simulink model "MIMO_FLOATING_POINT"  (R2023b)
settings: Solver=VariableStepAuto  StartTime=0.0  StopTime=1000  RelTol=1e-3
libraries: dspsigops x80, commchan3 x4, commdigbbndpm3 x2, commfilt2 x2, commsink2 x1, simulink x1, commrandsrc3 x1
(part 1 of 3)
settings Model: Creator=pc1  LastModifiedBy=yousi
settings SolverCC: AlgebraicLoopSolver=TrustRegion
settings DataIOCC: SaveOutput=off  SignalLogging=off  DSMLogging=off  SaveTime=off  ReturnWorkspaceOutputs=off
settings DebuggingCC: ArithmeticOperatorsInVariantConditions=warning
settings ModelReferenceCC: EnableRefExpFcnMdlSchedulingChecks=on
settings SFSimCC: CustomCodeUndefinedFunction=UseInterfaceOnly
settings CodeAppCC: StateflowObjectComments=on

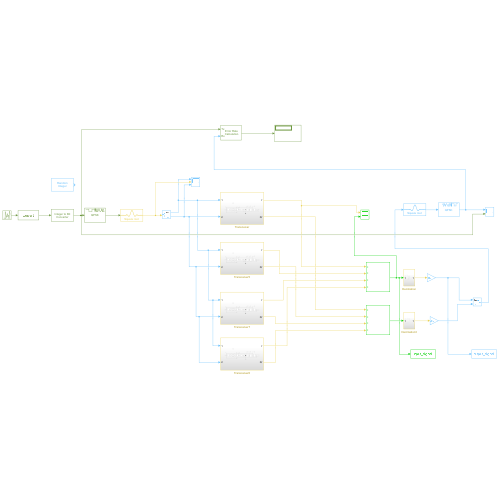
[thumbnail: Simulink's stored preview of the top-level diagram]
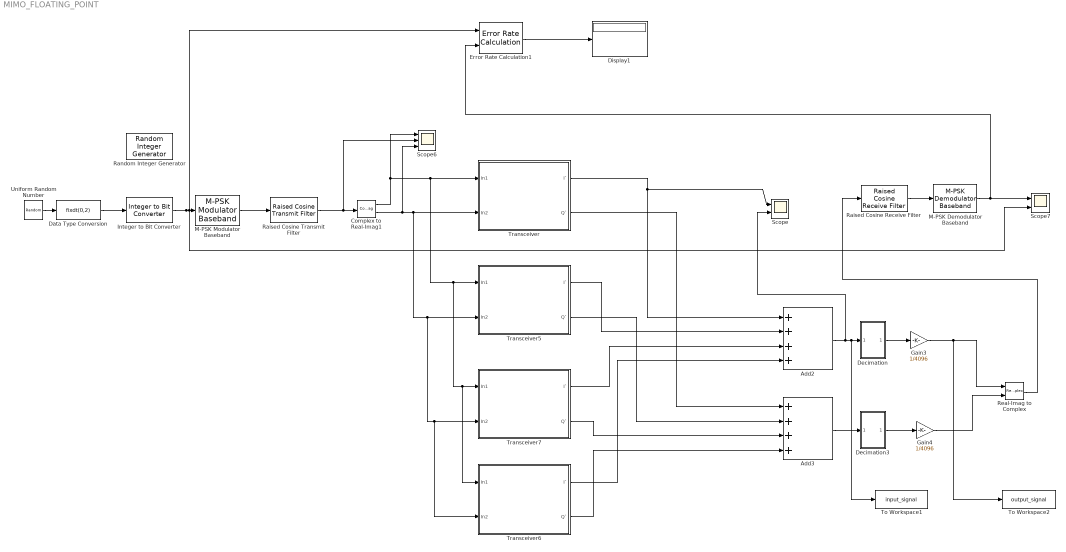
== system MIMO_FLOATING_POINT ==
  Add2 : Sum  Inputs=++++
  Add3 : Sum  Inputs=++++
  Complex to Real-Imag1 : ComplexToRealImag
  Data Type Conversion : DataTypeConversion  OutMin=0  OutMax=3  OutDataTypeStr=fixdt(0,2)  RndMeth=Round  SaturateOnIntegerOverflow=off
  Decimation : Subsystem
  Decimation3 : Subsystem
  Display1 : Display
  Error Rate Calculation1 : commsink2/Error Rate Calculation  N=28  st_delay=0  cp_mode=Entire frame  subframe=[]  PMode=Port  WsName=ErrorVec  RsMode2=off  stop=off  numErr=100  maxBits=1e6
  Gain3 : Gain  Gain=1/4096
  Gain4 : Gain  Gain=1/4096
  Integer to Bit Converter : simulink/Logic and Bit Operations/Integer to Bit Converter  nbits=2  signedInputValues=Unsigned  bitOrder=MSB first  outDtype=Inherit via internal rule
      settings: LibrarySourceBlock=|
      | commutil2/Integer to Bit
      | Converter
  M-PSK Demodulator Baseband : commdigbbndpm3/M-PSK Demodulator Baseband  M=4  OutType=Bit  DecType=Hard decision  VarSource=Dialog  Variance=1  Dec=Gray  Mapping=[0:7]  Ph=pi/4  outDtype1=Inherit via internal rule  outDtype2=Inherit via internal rule  derotateFactorWordLen=16  derotateFactorDataTypeStr=Inherit: Same word length as input  derotateFactorLastDataTypeStr=Inherit: Same word length as input
  M-PSK Modulator Baseband : commdigbbndpm3/M-PSK Modulator Baseband  M=4  InType=Bit  Enc=Gray  Mapping=[0:7]  Ph=pi/4  outDtype=double  outWordLen=16  outUDDataType=sfix(16)  outFracLenMode=Best precision  outFracLen=15  outDataTypeStr=double  outLastDataTypeStr=double
  Raised Cosine Receive Filter : commfilt2/Raised Cosine Receive Filter  filtType=Square root  R=0.35  filtSpan=8  N=2  downFactor=1  downOffset=0  filterGain=22  InputProcessing=Columns as channels (frame based)  RateOptions=Allow multirate processing  framing=Mute  checkCoeff=off  variableName=rcRxFilt  currentFiltSpan=10  D=5  inputOffset=0  sampMode=Mute  saveAsFlag=0  rateMode=Downsampling  checkGain=Normalized  launchFVT=on  roundingMode=Floor  overflowMode=off  coeffDataTypeStr=Inherit: Same word length as input  coeffMin=[]  coeffMax=[]  coeffLastDataTypeStr=Inherit: Same word length as input  accumDataTypeStr=Inherit: Same as product output  accumLastDataTypeStr=Inherit: Same as product output  outputDataTypeStr=Inherit: Same as accumulator  outputMin=[]  outputMax=[]  outputLastDataTypeStr=Inherit: Same as accumulator
  Raised Cosine Transmit Filter : commfilt2/Raised Cosine Transmit Filter  filtType=Square root  R=0.35  filtSpan=8  N=2  filterGain=22  InputProcessing=Columns as channels (frame based)  RateOptions=Allow multirate processing  framing=Mute  checkCoeff=off  variableName=rcTxFilt  checkGain=Normalized  sampMode=Mute  saveAsFlag=0  currentFiltSpan=10  D=5  launchFVT=on  roundingMode=Floor  overflowMode=off  coeffDataTypeStr=Inherit: Same word length as input  coeffMin=[]  coeffMax=[]  coeffLastDataTypeStr=Inherit: Same word length as input  outputDataTypeStr=Inherit: Same as accumulator  outputMin=[]  outputMax=[]  outputLastDataTypeStr=Inherit: Same as accumulator
  Random Integer Generator : commrandsrc3/Random Integer Generator  SetSize=2  SeedSource=Auto  Seed=0  SampleTime=0.64/4  SamplesPerFrame=2  OutputDataType=double  SimulateUsing=Interpreted execution
  Real-Imag to Complex : RealImagToComplex
  Scope : Scope  NumInputPorts=2
  Scope6 : Scope  NumInputPorts=3
  Scope7 : Scope  NumInputPorts=2
  To Workspace1 : ToWorkspace  VariableName=input_signal  SampleTime=-1
      settings: Save2DSignal=2-D array (concatenate along first dimension)
  To Workspace2 : ToWorkspace  VariableName=output_signal  SampleTime=-1
      settings: Save2DSignal=2-D array (concatenate along first dimension)
  Transceiver : Subsystem
  Transceiver5 : Subsystem
  Transceiver6 : Subsystem
  Transceiver7 : Subsystem
  Uniform Random Number : UniformRandomNumber  Minimum=0  Maximum=3  Seed=70  SampleTime=0.64
  wires:
  Integer to Bit Converter/1 -> Scope7/2, Error Rate Calculation1/1, M-PSK Modulator Baseband/1
  Gain3/1 -> To Workspace2/1, Real-Imag to Complex/1
  Transceiver/1(I`) -> Add2/1, Scope/1
  Raised Cosine Receive Filter/1 -> M-PSK Demodulator Baseband/1
  Add3/1 -> Decimation3/1(In1)
  Add2/1 -> Scope/2, To Workspace1/1, Decimation/1(In1)
  Transceiver6/2(Q`) -> Add3/4
  Transceiver6/1(I`) -> Add2/4
  Gain4/1 -> Real-Imag to Complex/2
  Transceiver7/1(I`) -> Add2/3
  Decimation3/1(Out1) -> Gain4/1
  Complex to Real-Imag1/1 -> Transceiver6/1(In1), Transceiver7/1(In1), Transceiver5/1(In1), Transceiver/1(In1), Scope6/1
  Uniform Random Number/1 -> Data Type Conversion/1
  Decimation/1(Out1) -> Gain3/1
  M-PSK Modulator Baseband/1 -> Raised Cosine Transmit Filter/1
  Transceiver5/2(Q`) -> Add3/2
  Transceiver/2(Q`) -> Add3/1
  Raised Cosine Transmit Filter/1 -> Complex to Real-Imag1/1, Scope6/2
  Transceiver5/1(I`) -> Add2/2
  Real-Imag to Complex/1 -> Raised Cosine Receive Filter/1
  M-PSK Demodulator Baseband/1 -> Scope7/1, Error Rate Calculation1/2
  Data Type Conversion/1 -> Integer to Bit Converter/1
  Complex to Real-Imag1/2 -> Transceiver6/2(In2), Transceiver7/2(In2), Transceiver5/2(In2), Transceiver/2(In2), Scope6/3
  Transceiver7/2(Q`) -> Add3/3
  Error Rate Calculation1/1 -> Display1/1

== system MIMO_FLOATING_POINT/Decimation ==
  In1 : Inport
  Add1 : Sum
  Delay{7..10,12..15} (8 alike) : Delay  DelayLength=1
  Downsample{,1..3,6..9} (8 alike) : DownSample  N=8  RateOptions=Allow multirate processing
  Downsample4 : DownSample  RateOptions=Allow multirate processing
  Downsample5 : DownSample  RateOptions=Allow multirate processing
  E0(Z)1 : Subsystem
  E1(Z)1 : Subsystem
  E10 : Subsystem
  E11 : Subsystem
  E12 : Subsystem
  E13 : Subsystem
  E14 : Subsystem
  E15 : Subsystem
  E8 : Subsystem
  E9 : Subsystem
  Gain1 : Gain  Gain=1/4096
  Sum3 : Sum  Inputs=|++++++++
  Out1 : Outport
  wires:
  Sum3/1 -> Gain1/1
  Downsample3/1 -> E11/1(In1)
  Delay7/1 -> Delay8/1, Downsample1/1
  Delay14/1 -> Delay15/1, Downsample8/1
  E13/1(Out1) -> Sum3/6
  E10/1(Out1) -> Sum3/3
  Downsample6/1 -> E12/1(In1)
  E14/1(Out1) -> Sum3/7
  E15/1(Out1) -> Sum3/8
  Delay9/1 -> Delay12/1, Downsample3/1
  E8/1(Out1) -> Sum3/1
  Delay10/1 -> Downsample5/1
  Downsample/1 -> E8/1(In1)
  Gain1/1 -> Downsample4/1, Delay10/1
  E11/1(Out1) -> Sum3/4
  Delay12/1 -> Delay13/1, Downsample6/1
  E9/1(Out1) -> Sum3/2
  In1/1 -> Delay7/1, Downsample/1
  Downsample8/1 -> E14/1(In1)
  E0(Z)1/1(Out1) -> Add1/1
  Delay13/1 -> Delay14/1, Downsample7/1
  Delay15/1 -> Downsample9/1
  Add1/1 -> Out1/1
  Downsample7/1 -> E13/1(In1)
  Delay8/1 -> Delay9/1, Downsample2/1
  Downsample2/1 -> E10/1(In1)
  Downsample4/1 -> E0(Z)1/1(Input)
  Downsample5/1 -> E1(Z)1/1(Input1)
  E12/1(Out1) -> Sum3/5
  E1(Z)1/1(Output) -> Add1/2
  Downsample1/1 -> E9/1(In1)
  Downsample9/1 -> E15/1(In1)

== system MIMO_FLOATING_POINT/Decimation3 ==
  In1 : Inport
  Add1 : Sum
  Delay{7..10,12..15} (8 alike) : Delay  DelayLength=1
  Downsample{,1..3,6..9} (8 alike) : DownSample  N=8  RateOptions=Allow multirate processing
  Downsample4 : DownSample  RateOptions=Allow multirate processing
  Downsample5 : DownSample  RateOptions=Allow multirate processing
  E0(Z)1 : Subsystem
  E1(Z)1 : Subsystem
  E10 : Subsystem
  E11 : Subsystem
  E12 : Subsystem
  E13 : Subsystem
  E14 : Subsystem
  E15 : Subsystem
  E8 : Subsystem
  E9 : Subsystem
  Gain1 : Gain  Gain=1/4096
  Sum3 : Sum  Inputs=|++++++++
  Out1 : Outport
  wires:
  Sum3/1 -> Gain1/1
  Downsample3/1 -> E11/1(In1)
  Delay7/1 -> Delay8/1, Downsample1/1
  Delay14/1 -> Delay15/1, Downsample8/1
  E13/1(Out1) -> Sum3/6
  E10/1(Out1) -> Sum3/3
  Downsample6/1 -> E12/1(In1)
  E14/1(Out1) -> Sum3/7
  E15/1(Out1) -> Sum3/8
  Delay9/1 -> Delay12/1, Downsample3/1
  E8/1(Out1) -> Sum3/1
  Delay10/1 -> Downsample5/1
  Downsample/1 -> E8/1(In1)
  Gain1/1 -> Downsample4/1, Delay10/1
  E11/1(Out1) -> Sum3/4
  Delay12/1 -> Delay13/1, Downsample6/1
  E9/1(Out1) -> Sum3/2
  In1/1 -> Delay7/1, Downsample/1
  Downsample8/1 -> E14/1(In1)
  E0(Z)1/1(Out1) -> Add1/1
  Delay13/1 -> Delay14/1, Downsample7/1
  Delay15/1 -> Downsample9/1
  Add1/1 -> Out1/1
  Downsample7/1 -> E13/1(In1)
  Delay8/1 -> Delay9/1, Downsample2/1
  Downsample2/1 -> E10/1(In1)
  Downsample4/1 -> E0(Z)1/1(Input)
  Downsample5/1 -> E1(Z)1/1(Input1)
  E12/1(Out1) -> Sum3/5
  E1(Z)1/1(Output) -> Add1/2
  Downsample1/1 -> E9/1(In1)
  Downsample9/1 -> E15/1(In1)

== system MIMO_FLOATING_POINT/Transceiver ==
  In1 : Inport
  In2 : Inport  Port=2
  ADC 1 : Subsystem
  AWGN Channel : commchan3/AWGN Channel  noiseMode="Signal to noise ratio  (SNR)"  EbNodB=10  EsNodB=10  SNRdB=22  bitsPerSym=1  Ps=1  Tsym=(1.000000e-02 * 1)  variance=0.0001  seed=67  InputProcessing=Columns as channels (frame based)
  CWM_RX2 : Subsystem
  CWM_TX_Chain_1 : Subsystem
  Constant2 : Constant  Value=0
  DDC2 : Subsystem
  DUC2 : Subsystem
  Gain : Gain  Gain=1/32
  Gain1 : Gain  Gain=1/256
  Gain2 : Gain  Gain=1/256
  Inter_Lever2 : Subsystem
  "Interpolation " : Subsystem
  Interpolation 1 : Subsystem
  Scope{,1..2,4,8} (5 alike) : Scope
  Scope3 : Scope  NumInputPorts=2
  Scope5 : Scope  NumInputPorts=2
  Sine Wave : Sin  Frequency=2*pi*25  Phase=pi/2  SampleTime=0.01*2
  Sine Wave1 : Sin  Frequency=2*pi*25  SampleTime=0.01*2
  Subsystem : Subsystem
  Subsystem1 : Subsystem
  I` : Outport
  Q` : Outport  Port=2
  wires:
  Inter_Lever2/2(EVEN_Q) -> DDC2/2(EVEN_Q)
  DUC2/1(Out2) -> Gain/1, Scope1/1
  CWM_TX_Chain_1/2(Q_1) -> Interpolation 1/1(Input)
  AWGN Channel/1 -> Scope3/1, ADC 1/1(In1)
  Constant2/1 -> CWM_TX_Chain_1/1(PHI), CWM_RX2/1(In1)
  Gain/1 -> AWGN Channel/1
  CWM_TX_Chain_1/1(I_1) -> "Interpolation "/1(Input)
  Inter_Lever2/1(ODD_I) -> DDC2/1(ODD_I), Scope4/1
  ADC 1/1(bits 1&0) -> Inter_Lever2/1(bits 1&0), Scope2/1, Scope3/2
  CWM_RX2/1(I`) -> Scope5/1, I`/1
  DDC2/1(I_DDC) -> CWM_RX2/2(I_DDC), Scope8/1
  DDC2/2(Q_DDC) -> CWM_RX2/3(Q_DDC)
  In1/1 -> CWM_TX_Chain_1/2(Processor_I), Scope5/2
  In2/1 -> CWM_TX_Chain_1/3(Processor_Q)
  Subsystem/1(Out1) -> DUC2/1(I_1), Scope/1
  Subsystem1/1(Out1) -> DUC2/2(Q_1)
  "Interpolation "/1(Out1) -> Gain1/1
  Interpolation 1/1(Out1) -> Gain2/1
  Gain1/1 -> Subsystem/1(In1)
  Gain2/1 -> Subsystem1/1(In1)
  CWM_RX2/2(Q`) -> Q`/1

== system MIMO_FLOATING_POINT/Transceiver5 ==
  In1 : Inport
  In2 : Inport  Port=2
  ADC 1 : Subsystem
  AWGN Channel : commchan3/AWGN Channel  noiseMode="Signal to noise ratio  (SNR)"  EbNodB=10  EsNodB=10  SNRdB=22  bitsPerSym=1  Ps=1  Tsym=(1.000000e-02 * 1)  variance=0.0001  seed=67  InputProcessing=Columns as channels (frame based)
  CWM_RX2 : Subsystem
  CWM_TX_Chain_1 : Subsystem
  Constant2 : Constant  Value=0.8131
  DDC2 : Subsystem
  DUC2 : Subsystem
  Gain : Gain  Gain=1/32
  Gain1 : Gain  Gain=1/256
  Gain2 : Gain  Gain=1/256
  Inter_Lever2 : Subsystem
  "Interpolation " : Subsystem
  Interpolation 1 : Subsystem
  Scope{,1..2,4,8} (5 alike) : Scope
  Scope3 : Scope  NumInputPorts=2
  Scope5 : Scope  NumInputPorts=2
  Sine Wave : Sin  Frequency=2*pi*25  Phase=pi/2  SampleTime=0.01*2
  Sine Wave1 : Sin  Frequency=2*pi*25  SampleTime=0.01*2
  Subsystem : Subsystem
  Subsystem1 : Subsystem
  I` : Outport
  Q` : Outport  Port=2
  wires:
  Inter_Lever2/2(EVEN_Q) -> DDC2/2(EVEN_Q)
  DUC2/1(Out2) -> Gain/1, Scope1/1
  CWM_TX_Chain_1/2(Q_1) -> Interpolation 1/1(Input)
  AWGN Channel/1 -> Scope3/1, ADC 1/1(In1)
  Constant2/1 -> CWM_TX_Chain_1/1(PHI), CWM_RX2/1(In1)
  Gain/1 -> AWGN Channel/1
  CWM_TX_Chain_1/1(I_1) -> "Interpolation "/1(Input)
  Inter_Lever2/1(ODD_I) -> DDC2/1(ODD_I), Scope4/1
  ADC 1/1(bits 1&0) -> Inter_Lever2/1(bits 1&0), Scope2/1, Scope3/2
  CWM_RX2/1(I`) -> Scope5/1, I`/1
  DDC2/1(I_DDC) -> CWM_RX2/2(I_DDC), Scope8/1
  DDC2/2(Q_DDC) -> CWM_RX2/3(Q_DDC)
  In1/1 -> CWM_TX_Chain_1/2(Processor_I), Scope5/2
  In2/1 -> CWM_TX_Chain_1/3(Processor_Q)
  Subsystem/1(Out1) -> DUC2/1(I_1), Scope/1
  Subsystem1/1(Out1) -> DUC2/2(Q_1)
  "Interpolation "/1(Out1) -> Gain1/1
  Interpolation 1/1(Out1) -> Gain2/1
  Gain1/1 -> Subsystem/1(In1)
  Gain2/1 -> Subsystem1/1(In1)
  CWM_RX2/2(Q`) -> Q`/1

== system MIMO_FLOATING_POINT/Transceiver6 ==
  In1 : Inport
  In2 : Inport  Port=2
  ADC 1 : Subsystem
  AWGN Channel : commchan3/AWGN Channel  noiseMode="Signal to noise ratio  (SNR)"  EbNodB=10  EsNodB=10  SNRdB=22  bitsPerSym=1  Ps=1  Tsym=(1.000000e-02 * 1)  variance=0.0001  seed=67  InputProcessing=Columns as channels (frame based)
  CWM_RX2 : Subsystem
  CWM_TX_Chain_1 : Subsystem
  Constant2 : Constant  Value=2.4393
  DDC2 : Subsystem
  DUC2 : Subsystem
  Gain : Gain  Gain=1/32
  Gain1 : Gain  Gain=1/256
  Gain2 : Gain  Gain=1/256
  Inter_Lever2 : Subsystem
  "Interpolation " : Subsystem
  Interpolation 1 : Subsystem
  Scope{,1..2,4,8} (5 alike) : Scope
  Scope3 : Scope  NumInputPorts=2
  Scope5 : Scope  NumInputPorts=2
  Sine Wave : Sin  Frequency=2*pi*25  Phase=pi/2  SampleTime=0.01*2
  Sine Wave1 : Sin  Frequency=2*pi*25  SampleTime=0.01*2
  Subsystem : Subsystem
  Subsystem1 : Subsystem
  I` : Outport
  Q` : Outport  Port=2
  wires:
  Inter_Lever2/2(EVEN_Q) -> DDC2/2(EVEN_Q)
  DUC2/1(Out2) -> Gain/1, Scope1/1
  CWM_TX_Chain_1/2(Q_1) -> Interpolation 1/1(Input)
  AWGN Channel/1 -> Scope3/1, ADC 1/1(In1)
  Constant2/1 -> CWM_TX_Chain_1/1(PHI), CWM_RX2/1(In1)
  Gain/1 -> AWGN Channel/1
  CWM_TX_Chain_1/1(I_1) -> "Interpolation "/1(Input)
  Inter_Lever2/1(ODD_I) -> DDC2/1(ODD_I), Scope4/1
  ADC 1/1(bits 1&0) -> Inter_Lever2/1(bits 1&0), Scope2/1, Scope3/2
  CWM_RX2/1(I`) -> Scope5/1, I`/1
  DDC2/1(I_DDC) -> CWM_RX2/2(I_DDC), Scope8/1
  DDC2/2(Q_DDC) -> CWM_RX2/3(Q_DDC)
  In1/1 -> CWM_TX_Chain_1/2(Processor_I), Scope5/2
  In2/1 -> CWM_TX_Chain_1/3(Processor_Q)
  Subsystem/1(Out1) -> DUC2/1(I_1), Scope/1
  Subsystem1/1(Out1) -> DUC2/2(Q_1)
  "Interpolation "/1(Out1) -> Gain1/1
  Interpolation 1/1(Out1) -> Gain2/1
  Gain1/1 -> Subsystem/1(In1)
  Gain2/1 -> Subsystem1/1(In1)
  CWM_RX2/2(Q`) -> Q`/1

== system MIMO_FLOATING_POINT/Transceiver7 ==
  In1 : Inport
  In2 : Inport  Port=2
  ADC 1 : Subsystem
  AWGN Channel : commchan3/AWGN Channel  noiseMode="Signal to noise ratio  (SNR)"  EbNodB=10  EsNodB=10  SNRdB=22  bitsPerSym=1  Ps=1  Tsym=(1.000000e-02 * 1)  variance=0.0001  seed=67  InputProcessing=Columns as channels (frame based)
  CWM_RX2 : Subsystem
  CWM_TX_Chain_1 : Subsystem
  Constant2 : Constant  Value=1.6262
  DDC2 : Subsystem
  DUC2 : Subsystem
  Gain : Gain  Gain=1/32
  Gain1 : Gain  Gain=1/256
  Gain2 : Gain  Gain=1/256
  Inter_Lever2 : Subsystem
  "Interpolation " : Subsystem
  Interpolation 1 : Subsystem
  Scope{,1..2,4,8} (5 alike) : Scope
  Scope3 : Scope  NumInputPorts=2
  Scope5 : Scope  NumInputPorts=2
  Sine Wave : Sin  Frequency=2*pi*25  Phase=pi/2  SampleTime=0.01*2
  Sine Wave1 : Sin  Frequency=2*pi*25  SampleTime=0.01*2
  Subsystem : Subsystem
  Subsystem1 : Subsystem
  I` : Outport
  Q` : Outport  Port=2
  wires:
  Inter_Lever2/2(EVEN_Q) -> DDC2/2(EVEN_Q)
  DUC2/1(Out2) -> Gain/1, Scope1/1
  CWM_TX_Chain_1/2(Q_1) -> Interpolation 1/1(Input)
  AWGN Channel/1 -> Scope3/1, ADC 1/1(In1)
  Constant2/1 -> CWM_TX_Chain_1/1(PHI), CWM_RX2/1(In1)
  Gain/1 -> AWGN Channel/1
  CWM_TX_Chain_1/1(I_1) -> "Interpolation "/1(Input)
  Inter_Lever2/1(ODD_I) -> DDC2/1(ODD_I), Scope4/1
  ADC 1/1(bits 1&0) -> Inter_Lever2/1(bits 1&0), Scope2/1, Scope3/2
  CWM_RX2/1(I`) -> Scope5/1, I`/1
  DDC2/1(I_DDC) -> CWM_RX2/2(I_DDC), Scope8/1
  DDC2/2(Q_DDC) -> CWM_RX2/3(Q_DDC)
  In1/1 -> CWM_TX_Chain_1/2(Processor_I), Scope5/2
  In2/1 -> CWM_TX_Chain_1/3(Processor_Q)
  Subsystem/1(Out1) -> DUC2/1(I_1), Scope/1
  Subsystem1/1(Out1) -> DUC2/2(Q_1)
  "Interpolation "/1(Out1) -> Gain1/1
  Interpolation 1/1(Out1) -> Gain2/1
  Gain1/1 -> Subsystem/1(In1)
  Gain2/1 -> Subsystem1/1(In1)
  CWM_RX2/2(Q`) -> Q`/1

== system MIMO_FLOATING_POINT/Decimation/E0(Z)1 ==
  Input : Inport
  Delay : Delay  DelayLength=5
  Gain : Gain  Gain=0.5
  Out1 : Outport
  wires:
  Input/1 -> Gain/1
  Delay/1 -> Out1/1
  Gain/1 -> Delay/1

== system MIMO_FLOATING_POINT/Decimation/E1(Z)1 ==
  Input1 : Inport
  10-12 : Gain  Gain=0.3078
  2-20 : Gain  Gain=0.0011
  4-18 : Gain  Gain=-0.0072
  6-16 : Gain  Gain=0.0263
  8-14 : Gain  Gain=-0.078
  Add{7..10,12..16} (9 alike) : Sum
  Delay{21,23,25,27,29,31,33,35,37} (9 alike) : Delay  DelayLength=1
  Output : Outport
  wires:
  8-14/1 -> Add13/1, Add9/1
  Delay29/1 -> Add12/2  "x[n-11]"
  Add14/1 -> Delay35/1
  Input1/1 -> 2-20/1, 4-18/1, 6-16/1, 8-14/1, 10-12/1
  Add8/1 -> Delay25/1
  4-18/1 -> Add15/1, Add7/1
  Delay33/1 -> Add14/2  "x[n-15]"
  Add12/1 -> Delay31/1
  10-12/1 -> Add10/1, Add12/1
  Add9/1 -> Delay27/1
  Add16/1 -> Output/1
  Delay37/1 -> Add16/2  "x[n-19]"
  6-16/1 -> Add14/1, Add8/1
  Delay25/1 -> Add9/2  "x[n-7]"
  Add7/1 -> Delay23/1
  Add15/1 -> Delay37/1
  Delay23/1 -> Add8/2  "x[n-5]"
  Delay27/1 -> Add10/2  "x[n-9]"
  Delay31/1 -> Add13/2  "x[n-13]"
  Delay35/1 -> Add15/2  "x[n-17]"
  Delay21/1 -> Add7/2  "x[n-3]"
  2-20/1 -> Delay21/1, Add16/1
  Add13/1 -> Delay33/1
  Add10/1 -> Delay29/1

== system MIMO_FLOATING_POINT/Decimation/E10 ==
  In1 : Inport
  Delay3 : Delay  DelayLength=1
  Delay4 : Delay  DelayLength=1
  Delay5 : Delay  DelayLength=1
  Gain : Gain  Gain=10
  Gain1 : Gain  Gain=246
  Sum : Sum
  Sum1 : Sum
  Sum2 : Sum
  Out1 : Outport
  wires:
  In1/1 -> Gain1/1, Gain/1
  Sum1/1 -> Delay5/1
  Sum/1 -> Delay4/1
  Gain1/1 -> Sum1/1, Sum/1
  Delay3/1 -> Sum/2
  Delay4/1 -> Sum1/2
  Gain/1 -> Sum2/1, Delay3/1
  Delay5/1 -> Sum2/2
  Sum2/1 -> Out1/1

== system MIMO_FLOATING_POINT/Decimation/E11 ==
  In1 : Inport
  Delay3 : Delay  DelayLength=1
  Delay4 : Delay  DelayLength=1
  Delay5 : Delay  DelayLength=1
  Gain : Gain  Gain=4
  Gain1 : Gain  Gain=204
  Gain2 : Gain  Gain=284
  Gain3 : Gain  Gain=20
  Sum : Sum
  Sum1 : Sum
  Sum2 : Sum
  Out1 : Outport
  wires:
  In1/1 -> Gain2/1, Gain3/1, Gain1/1, Gain/1
  Sum1/1 -> Delay5/1
  Sum/1 -> Delay4/1
  Gain1/1 -> Sum/1
  Delay3/1 -> Sum/2
  Delay4/1 -> Sum1/2
  Gain3/1 -> Sum2/1
  Delay5/1 -> Sum2/2
  Gain/1 -> Delay3/1
  Sum2/1 -> Out1/1
  Gain2/1 -> Sum1/1

== system MIMO_FLOATING_POINT/Decimation/E12 ==
  In1 : Inport
  Delay3 : Delay  DelayLength=1
  Delay4 : Delay  DelayLength=1
  Delay5 : Delay  DelayLength=1
  Gain : Gain
  Gain1 : Gain  Gain=161
  Gain2 : Gain  Gain=315
  Gain3 : Gain  Gain=35
  Sum : Sum
  Sum1 : Sum
  Sum2 : Sum
  Out1 : Outport
  wires:
  In1/1 -> Gain2/1, Gain3/1, Gain1/1, Gain/1
  Sum1/1 -> Delay5/1
  Sum/1 -> Delay4/1
  Gain1/1 -> Sum/1
  Delay3/1 -> Sum/2
  Delay4/1 -> Sum1/2
  Gain3/1 -> Sum2/1
  Delay5/1 -> Sum2/2
  Gain/1 -> Delay3/1
  Sum2/1 -> Out1/1
  Gain2/1 -> Sum1/1

== system MIMO_FLOATING_POINT/Decimation/E13 ==
  In1 : Inport
  Delay6 : Delay  DelayLength=1
  Delay7 : Delay  DelayLength=1
  Gain4 : Gain  Gain=120
  Gain5 : Gain  Gain=336
  Gain6 : Gain  Gain=56
  Sum4 : Sum
  Sum5 : Sum
  Out1 : Outport
  wires:
  Gain4/1 -> Delay6/1
  In1/1 -> Gain6/1, Gain5/1, Gain4/1
  Sum5/1 -> Out1/1
  Sum4/1 -> Delay7/1
  Delay7/1 -> Sum5/2
  Gain6/1 -> Sum5/1
  Gain5/1 -> Sum4/1
  Delay6/1 -> Sum4/2

== system MIMO_FLOATING_POINT/Decimation/E14 ==
  In1 : Inport
  Delay6 : Delay  DelayLength=1
  Delay7 : Delay  DelayLength=1
  Gain4 : Gain  Gain=84
  Gain5 : Gain  Gain=344
  Sum4 : Sum
  Sum5 : Sum
  Out1 : Outport
  wires:
  In1/1 -> Gain5/1, Gain4/1
  Sum5/1 -> Out1/1
  Sum4/1 -> Delay7/1
  Delay7/1 -> Sum5/2
  Gain4/1 -> Sum5/1, Delay6/1
  Gain5/1 -> Sum4/1
  Delay6/1 -> Sum4/2

== system MIMO_FLOATING_POINT/Decimation/E15 ==
  In1 : Inport
  Delay6 : Delay  DelayLength=1
  Delay7 : Delay  DelayLength=1
  Gain4 : Gain  Gain=56
  Gain5 : Gain  Gain=336
  Gain6 : Gain  Gain=120
  Sum4 : Sum
  Sum5 : Sum
  Out1 : Outport
  wires:
  Gain4/1 -> Delay6/1
  In1/1 -> Gain6/1, Gain5/1, Gain4/1
  Sum5/1 -> Out1/1
  Sum4/1 -> Delay7/1
  Delay7/1 -> Sum5/2
  Gain6/1 -> Sum5/1
  Gain5/1 -> Sum4/1
  Delay6/1 -> Sum4/2

== system MIMO_FLOATING_POINT/Decimation/E8 ==
  In1 : Inport
  Delay3 : Delay  DelayLength=1
  Delay4 : Delay  DelayLength=1
  Delay5 : Delay  DelayLength=1
  Gain : Gain  Gain=35
  Gain1 : Gain  Gain=315
  Gain2 : Gain  Gain=161
  Gain3 : Gain
  Sum : Sum
  Sum1 : Sum
  Sum2 : Sum
  Out1 : Outport
  wires:
  In1/1 -> Gain2/1, Gain3/1, Gain1/1, Gain/1
  Sum1/1 -> Delay5/1
  Sum/1 -> Delay4/1
  Gain1/1 -> Sum/1
  Delay3/1 -> Sum/2
  Delay4/1 -> Sum1/2
  Gain3/1 -> Sum2/1
  Delay5/1 -> Sum2/2
  Gain/1 -> Delay3/1
  Sum2/1 -> Out1/1
  Gain2/1 -> Sum1/1

== system MIMO_FLOATING_POINT/Decimation/E9 ==
  In1 : Inport
  Delay3 : Delay  DelayLength=1
  Delay4 : Delay  DelayLength=1
  Delay5 : Delay  DelayLength=1
  Gain : Gain  Gain=20
  Gain1 : Gain  Gain=284
  Gain2 : Gain  Gain=204
  Gain3 : Gain  Gain=4
  Sum : Sum
  Sum1 : Sum
  Sum2 : Sum
  Out1 : Outport
  wires:
  In1/1 -> Gain2/1, Gain3/1, Gain1/1, Gain/1
  Sum1/1 -> Delay5/1
  Sum/1 -> Delay4/1
  Gain1/1 -> Sum/1
  Delay3/1 -> Sum/2
  Delay4/1 -> Sum1/2
  Gain3/1 -> Sum2/1
  Delay5/1 -> Sum2/2
  Gain/1 -> Delay3/1
  Sum2/1 -> Out1/1
  Gain2/1 -> Sum1/1

== system MIMO_FLOATING_POINT/Decimation3/E0(Z)1 ==
  Input : Inport
  Delay : Delay  DelayLength=5
  Gain : Gain  Gain=0.5
  Out1 : Outport
  wires:
  Input/1 -> Gain/1
  Delay/1 -> Out1/1
  Gain/1 -> Delay/1

== system MIMO_FLOATING_POINT/Decimation3/E1(Z)1 ==
  Input1 : Inport
  10-12 : Gain  Gain=0.3078
  2-20 : Gain  Gain=0.0011
  4-18 : Gain  Gain=-0.0072
  6-16 : Gain  Gain=0.0263
  8-14 : Gain  Gain=-0.078
  Add{7..10,12..16} (9 alike) : Sum
  Delay{21,23,25,27,29,31,33,35,37} (9 alike) : Delay  DelayLength=1
  Output : Outport
  wires:
  8-14/1 -> Add13/1, Add9/1
  Delay29/1 -> Add12/2  "x[n-11]"
  Add14/1 -> Delay35/1
  Input1/1 -> 2-20/1, 4-18/1, 6-16/1, 8-14/1, 10-12/1
  Add8/1 -> Delay25/1
  4-18/1 -> Add15/1, Add7/1
  Delay33/1 -> Add14/2  "x[n-15]"
  Add12/1 -> Delay31/1
  10-12/1 -> Add10/1, Add12/1
  Add9/1 -> Delay27/1
  Add16/1 -> Output/1
  Delay37/1 -> Add16/2  "x[n-19]"
  6-16/1 -> Add14/1, Add8/1
  Delay25/1 -> Add9/2  "x[n-7]"
  Add7/1 -> Delay23/1
  Add15/1 -> Delay37/1
  Delay23/1 -> Add8/2  "x[n-5]"
  Delay27/1 -> Add10/2  "x[n-9]"
  Delay31/1 -> Add13/2  "x[n-13]"
  Delay35/1 -> Add15/2  "x[n-17]"
  Delay21/1 -> Add7/2  "x[n-3]"
  2-20/1 -> Delay21/1, Add16/1
  Add13/1 -> Delay33/1
  Add10/1 -> Delay29/1

== system MIMO_FLOATING_POINT/Decimation3/E10 ==
  In1 : Inport
  Delay3 : Delay  DelayLength=1
  Delay4 : Delay  DelayLength=1
  Delay5 : Delay  DelayLength=1
  Gain : Gain  Gain=10
  Gain1 : Gain  Gain=246
  Sum : Sum
  Sum1 : Sum
  Sum2 : Sum
  Out1 : Outport
  wires:
  In1/1 -> Gain1/1, Gain/1
  Sum1/1 -> Delay5/1
  Sum/1 -> Delay4/1
  Gain1/1 -> Sum1/1, Sum/1
  Delay3/1 -> Sum/2
  Delay4/1 -> Sum1/2
  Gain/1 -> Sum2/1, Delay3/1
  Delay5/1 -> Sum2/2
  Sum2/1 -> Out1/1

== system MIMO_FLOATING_POINT/Decimation3/E11 ==
  In1 : Inport
  Delay3 : Delay  DelayLength=1
  Delay4 : Delay  DelayLength=1
  Delay5 : Delay  DelayLength=1
  Gain : Gain  Gain=4
  Gain1 : Gain  Gain=204
  Gain2 : Gain  Gain=284
  Gain3 : Gain  Gain=20
  Sum : Sum
  Sum1 : Sum
  Sum2 : Sum
  Out1 : Outport
  wires:
  In1/1 -> Gain2/1, Gain3/1, Gain1/1, Gain/1
  Sum1/1 -> Delay5/1
  Sum/1 -> Delay4/1
  Gain1/1 -> Sum/1
  Delay3/1 -> Sum/2
  Delay4/1 -> Sum1/2
  Gain3/1 -> Sum2/1
  Delay5/1 -> Sum2/2
  Gain/1 -> Delay3/1
  Sum2/1 -> Out1/1
  Gain2/1 -> Sum1/1

== system MIMO_FLOATING_POINT/Decimation3/E12 ==
  In1 : Inport
  Delay3 : Delay  DelayLength=1
  Delay4 : Delay  DelayLength=1
  Delay5 : Delay  DelayLength=1
  Gain : Gain
  Gain1 : Gain  Gain=161
  Gain2 : Gain  Gain=315
  Gain3 : Gain  Gain=35
  Sum : Sum
  Sum1 : Sum
  Sum2 : Sum
  Out1 : Outport
  wires:
  In1/1 -> Gain2/1, Gain3/1, Gain1/1, Gain/1
  Sum1/1 -> Delay5/1
  Sum/1 -> Delay4/1
  Gain1/1 -> Sum/1
  Delay3/1 -> Sum/2
  Delay4/1 -> Sum1/2
  Gain3/1 -> Sum2/1
  Delay5/1 -> Sum2/2
  Gain/1 -> Delay3/1
  Sum2/1 -> Out1/1
  Gain2/1 -> Sum1/1

== system MIMO_FLOATING_POINT/Decimation3/E13 ==
  In1 : Inport
  Delay6 : Delay  DelayLength=1
  Delay7 : Delay  DelayLength=1
  Gain4 : Gain  Gain=120
  Gain5 : Gain  Gain=336
  Gain6 : Gain  Gain=56
  Sum4 : Sum
  Sum5 : Sum
  Out1 : Outport
  wires:
  Gain4/1 -> Delay6/1
  In1/1 -> Gain6/1, Gain5/1, Gain4/1
  Sum5/1 -> Out1/1
  Sum4/1 -> Delay7/1
  Delay7/1 -> Sum5/2
  Gain6/1 -> Sum5/1
  Gain5/1 -> Sum4/1
  Delay6/1 -> Sum4/2

== system MIMO_FLOATING_POINT/Decimation3/E14 ==
  In1 : Inport
  Delay6 : Delay  DelayLength=1
  Delay7 : Delay  DelayLength=1
  Gain4 : Gain  Gain=84
  Gain5 : Gain  Gain=344
  Sum4 : Sum
  Sum5 : Sum
  Out1 : Outport
  wires:
  In1/1 -> Gain5/1, Gain4/1
  Sum5/1 -> Out1/1
  Sum4/1 -> Delay7/1
  Delay7/1 -> Sum5/2
  Gain4/1 -> Sum5/1, Delay6/1
  Gain5/1 -> Sum4/1
  Delay6/1 -> Sum4/2

== system MIMO_FLOATING_POINT/Decimation3/E15 ==
  In1 : Inport
  Delay6 : Delay  DelayLength=1
  Delay7 : Delay  DelayLength=1
  Gain4 : Gain  Gain=56
  Gain5 : Gain  Gain=336
  Gain6 : Gain  Gain=120
  Sum4 : Sum
  Sum5 : Sum
  Out1 : Outport
  wires:
  Gain4/1 -> Delay6/1
  In1/1 -> Gain6/1, Gain5/1, Gain4/1
  Sum5/1 -> Out1/1
  Sum4/1 -> Delay7/1
  Delay7/1 -> Sum5/2
  Gain6/1 -> Sum5/1
  Gain5/1 -> Sum4/1
  Delay6/1 -> Sum4/2

== system MIMO_FLOATING_POINT/Decimation3/E8 ==
  In1 : Inport
  Delay3 : Delay  DelayLength=1
  Delay4 : Delay  DelayLength=1
  Delay5 : Delay  DelayLength=1
  Gain : Gain  Gain=35
  Gain1 : Gain  Gain=315
  Gain2 : Gain  Gain=161
  Gain3 : Gain
  Sum : Sum
  Sum1 : Sum
  Sum2 : Sum
  Out1 : Outport
  wires:
  In1/1 -> Gain2/1, Gain3/1, Gain1/1, Gain/1
  Sum1/1 -> Delay5/1
  Sum/1 -> Delay4/1
  Gain1/1 -> Sum/1
  Delay3/1 -> Sum/2
  Delay4/1 -> Sum1/2
  Gain3/1 -> Sum2/1
  Delay5/1 -> Sum2/2
  Gain/1 -> Delay3/1
  Sum2/1 -> Out1/1
  Gain2/1 -> Sum1/1

== system MIMO_FLOATING_POINT/Decimation3/E9 ==
  In1 : Inport
  Delay3 : Delay  DelayLength=1
  Delay4 : Delay  DelayLength=1
  Delay5 : Delay  DelayLength=1
  Gain : Gain  Gain=20
  Gain1 : Gain  Gain=284
  Gain2 : Gain  Gain=204
  Gain3 : Gain  Gain=4
  Sum : Sum
  Sum1 : Sum
  Sum2 : Sum
  Out1 : Outport
  wires:
  In1/1 -> Gain2/1, Gain3/1, Gain1/1, Gain/1
  Sum1/1 -> Delay5/1
  Sum/1 -> Delay4/1
  Gain1/1 -> Sum/1
  Delay3/1 -> Sum/2
  Delay4/1 -> Sum1/2
  Gain3/1 -> Sum2/1
  Delay5/1 -> Sum2/2
  Gain/1 -> Delay3/1
  Sum2/1 -> Out1/1
  Gain2/1 -> Sum1/1

== system MIMO_FLOATING_POINT/Transceiver/ADC 1 ==
  In1 : Inport
  SigmaDelta ADC : Subsystem
  Switch : Switch  Criteria=u2 > Threshold  SaturateOnIntegerOverflow=off  InputSameDT=off
  Zero : Constant  Value=0
  bits 1&0 : Outport
  wires:
  SigmaDelta ADC/1(Out) -> Switch/1, Switch/2
  Zero/1 -> Switch/3
  In1/1 -> SigmaDelta ADC/1(In)
  Switch/1 -> bits 1&0/1

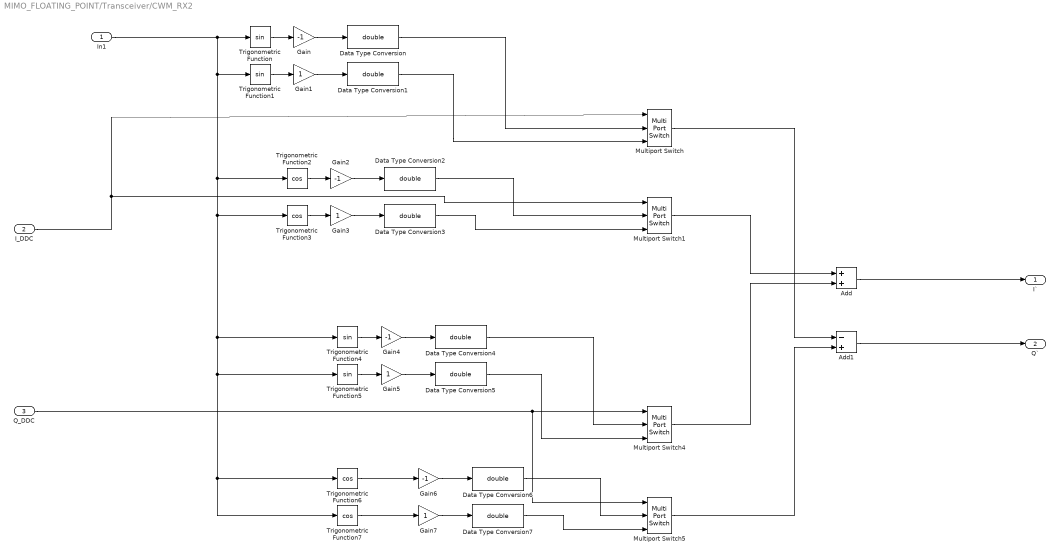
== system MIMO_FLOATING_POINT/Transceiver/CWM_RX2 ==
  In1 : Inport
  I_DDC : Inport  Port=2
  Q_DDC : Inport  Port=3
  Add : Sum
  Add1 : Sum  Inputs=-+
  Data Type Conversion{,1..7} (8 alike) : DataTypeConversion  OutMin=-1  OutMax=1  OutDataTypeStr=double  RndMeth=Nearest
  Gain{,2,4,6} (4 alike) : Gain  Gain=-1
  Gain{1,3,5,7} (4 alike) : Gain
  Multiport Switch{,1,4..5} (4 alike) : MultiPortSwitch  DataPortOrder=Zero-based contiguous  Inputs=2  zeroidx=on  RndMeth=Nearest  SaturateOnIntegerOverflow=off  InputSameDT=off
  Trigonometric Function{,1,4..5} (4 alike) : Trigonometry
  Trigonometric Function{2..3,6..7} (4 alike) : Trigonometry  Operator=cos
  I` : Outport
  Q` : Outport  Port=2
  wires:
  Multiport Switch/1 -> Add1/1
  Add/1 -> I`/1
  I_DDC/1 -> Multiport Switch1/1, Multiport Switch/1
  Gain2/1 -> Data Type Conversion2/1
  Trigonometric Function5/1 -> Gain5/1
  Data Type Conversion2/1 -> Multiport Switch1/2
  Data Type Conversion1/1 -> Multiport Switch/3
  Gain5/1 -> Data Type Conversion5/1
  Gain4/1 -> Data Type Conversion4/1
  Trigonometric Function1/1 -> Gain1/1
  Data Type Conversion6/1 -> Multiport Switch5/2
  Gain1/1 -> Data Type Conversion1/1
  Gain3/1 -> Data Type Conversion3/1
  Trigonometric Function3/1 -> Gain3/1
  Add1/1 -> Q`/1
  Gain/1 -> Data Type Conversion/1
  Trigonometric Function2/1 -> Gain2/1
  In1/1 -> Trigonometric Function3/1, Trigonometric Function4/1, Trigonometric Function5/1, Trigonometric Function6/1, Trigonometric Function7/1, Trigonometric Function2/1, Trigonometric Function1/1, Trigonometric Function/1
  Q_DDC/1 -> Multiport Switch5/1, Multiport Switch4/1
  Data Type Conversion7/1 -> Multiport Switch5/3
  Data Type Conversion4/1 -> Multiport Switch4/2
  Trigonometric Function6/1 -> Gain6/1
  Gain7/1 -> Data Type Conversion7/1
  Trigonometric Function4/1 -> Gain4/1
  Trigonometric Function/1 -> Gain/1
  Multiport Switch1/1 -> Add/1
  Multiport Switch4/1 -> Add/2
  Trigonometric Function7/1 -> Gain7/1
  Multiport Switch5/1 -> Add1/2
  Data Type Conversion5/1 -> Multiport Switch4/3
  Gain6/1 -> Data Type Conversion6/1
  Data Type Conversion/1 -> Multiport Switch/2
  Data Type Conversion3/1 -> Multiport Switch1/3

== system MIMO_FLOATING_POINT/Transceiver/CWM_TX_Chain_1 ==
  PHI : Inport
  Processor_I : Inport  Port=2
  Processor_Q : Inport  Port=3
  Add : Sum  OutDataTypeStr=double  RndMeth=Round  SaturateOnIntegerOverflow=on
  Add1 : Sum  OutDataTypeStr=double
  Data Type Conversion{1..4} (4 alike) : DataTypeConversion  Commented=through  OutMin=-1  OutMax=1  OutDataTypeStr=fixdt(1,8,6)  RndMeth=Nearest
  Gain1 : Gain  Gain=-1
  Gain2 : Gain
  Gain3 : Gain
  Gain4 : Gain
  Hamming : Gain  OutDataTypeStr=double
  Hamming1 : Gain  OutDataTypeStr=double
  Product{,1..3} (4 alike) : Product
  Trigonometric Function1 : Trigonometry
  Trigonometric Function2 : Trigonometry  Operator=cos
  Trigonometric Function3 : Trigonometry  Operator=cos
  Trigonometric Function4 : Trigonometry
  I_1 : Outport
  Q_1 : Outport  Port=2
  wires:
  Trigonometric Function2/1 -> Gain2/1
  Gain2/1 -> Data Type Conversion2/1
  Processor_Q/1 -> Product1/2, Product3/2
  Processor_I/1 -> Product2/1, Product/1
  Gain1/1 -> Data Type Conversion1/1
  Product/1 -> Add/1
  Trigonometric Function1/1 -> Gain1/1
  PHI/1 -> Trigonometric Function2/1, Trigonometric Function1/1, Trigonometric Function4/1, Trigonometric Function3/1
  Data Type Conversion1/1 -> Product1/1
  Gain3/1 -> Data Type Conversion3/1
  Product2/1 -> Add1/1
  Data Type Conversion2/1 -> Product/2
  Data Type Conversion4/1 -> Product2/2
  Data Type Conversion3/1 -> Product3/1
  Product3/1 -> Add1/2
  Trigonometric Function3/1 -> Gain3/1
  Product1/1 -> Add/2
  Gain4/1 -> Data Type Conversion4/1
  Trigonometric Function4/1 -> Gain4/1
  Add/1 -> Hamming/1
  Add1/1 -> Hamming1/1
  Hamming/1 -> I_1/1
  Hamming1/1 -> Q_1/1

== system MIMO_FLOATING_POINT/Transceiver/DDC2 ==
  ODD_I : Inport
  EVEN_Q : Inport  Port=2
  Local_Oscilator1 : DiscretePulseGenerator  PhaseDelay=1  SampleTime=0.02
  Logical Operator : Logic  Operator=NXOR  AllPortsSameDT=off  OutDataTypeStr=boolean
  Logical Operator1 : Logic  Operator=NXOR  AllPortsSameDT=off  OutDataTypeStr=boolean
  NOT : Logic  Operator=NOT  IconShape=distinctive  AllPortsSameDT=off  OutDataTypeStr=boolean
  Scope1 : Scope  NumInputPorts=3
  Scope2 : Scope  NumInputPorts=3
  I_DDC : Outport
  Q_DDC : Outport  Port=2
  wires:
  Logical Operator/1 -> Scope2/3, I_DDC/1
  EVEN_Q/1 -> Scope1/1, Logical Operator1/2
  ODD_I/1 -> Scope2/1, Logical Operator/1
  Logical Operator1/1 -> Scope1/3, Q_DDC/1
  Local_Oscilator1/1 -> NOT/1
  NOT/1 -> Scope1/2, Logical Operator1/1, Scope2/2, Logical Operator/2

== system MIMO_FLOATING_POINT/Transceiver/DUC2 ==
  I_1 : Inport
  Q_1 : Inport  Port=2
  -cos : Sin  SineType=Sample based  Frequency=2*pi*100  Phase=pi/2  Samples=4  SampleTime=0.01  Offset=3
  -sin1 : Sin  SineType=Sample based  Frequency=(2*pi*100)/4  Samples=4  SampleTime=.01  Offset=2
  Add : Sum
  Constant : Constant  Value=0
  Constant1 : Constant  Value=0
  Gain : Gain  Gain=-1
  Gain1 : Gain  Gain=-1
  Multiport Switch : MultiPortSwitch  DataPortOrder=Specify indices  DataPortIndices={1,0,-1}  RndMeth=Nearest  SaturateOnIntegerOverflow=off  InputSameDT=off
  Multiport Switch1 : MultiPortSwitch  DataPortOrder=Specify indices  DataPortIndices={1,0,-1}  RndMeth=Nearest  SaturateOnIntegerOverflow=off  InputSameDT=off
  Scope : Scope  NumInputPorts=3
  Scope1 : Scope  NumInputPorts=3
  Scope2 : Scope  NumInputPorts=3
  Out2 : Outport
  wires:
  Constant/1 -> Multiport Switch1/3
  Q_1/1 -> Gain1/1, Multiport Switch/2, Scope/1
  I_1/1 -> Gain/1, Scope2/1, Multiport Switch1/2
  Gain1/1 -> Multiport Switch/4
  -sin1/1 -> Scope/2, Multiport Switch/1
  -cos/1 -> Scope2/2, Multiport Switch1/1
  Multiport Switch/1 -> Scope/3, Scope1/2, Add/2
  Add/1 -> Scope1/3, Out2/1
  Multiport Switch1/1 -> Add/1, Scope1/1, Scope2/3
  Constant1/1 -> Multiport Switch/3
  Gain/1 -> Multiport Switch1/4

== system MIMO_FLOATING_POINT/Transceiver/Inter_Lever2 ==
  bits 1&0 : Inport
  Delay1 : Delay  DelayLength=1  InitialCondition=0
  Delay2 : Delay  DelayLength=1  InitialCondition=0
  Downsample : DownSample  RateOptions=Allow multirate processing
  Downsample1 : DownSample  RateOptions=Allow multirate processing
  Scope1 : Scope  NumInputPorts=3
  ODD_I : Outport
  EVEN_Q : Outport  Port=2
  wires:
  Delay1/1 -> Downsample1/1
  Downsample/1 -> Delay2/1
  Downsample1/1 -> Scope1/3, EVEN_Q/1
  bits 1&0/1 -> Scope1/1, Delay1/1, Downsample/1
  Delay2/1 -> Scope1/2, ODD_I/1

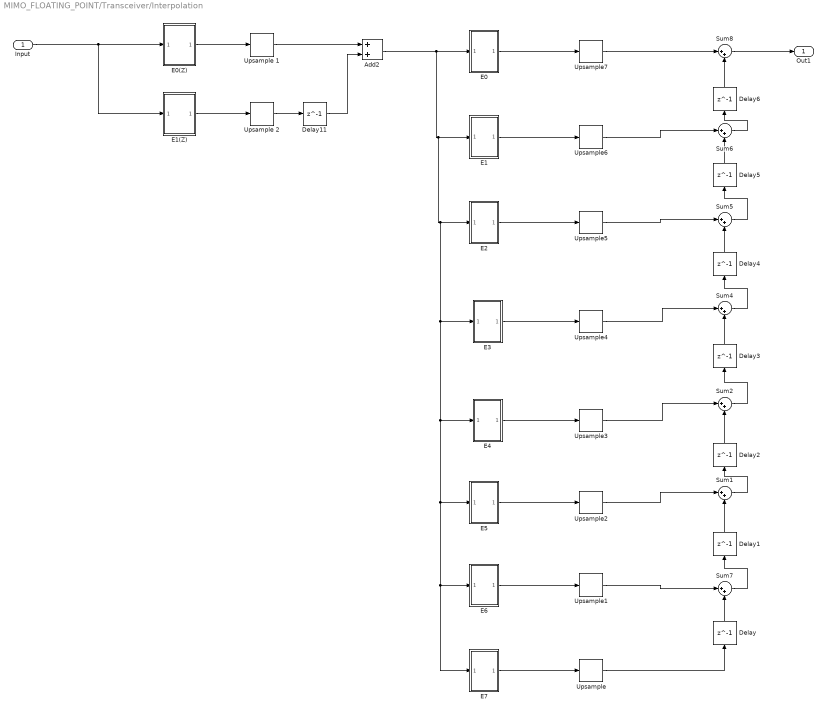
== system MIMO_FLOATING_POINT/Transceiver/Interpolation  ==
  Input : Inport
  Add2 : Sum
  Delay{,1..6,11} (8 alike) : Delay  DelayLength=1
  E0 : Subsystem
  E0(Z) : Subsystem
  E1 : Subsystem
  E1(Z) : Subsystem
  E2 : Subsystem
  E3 : Subsystem
  E4 : Subsystem
  E5 : Subsystem
  E6 : Subsystem
  E7 : Subsystem
  Sum{1..2,4..8} (7 alike) : Sum  Inputs=|++
  Upsample{,1..7} (8 alike) : dspsigops/Upsample  N=8  phase=0  RateOptions=Allow multirate processing  ic=0  mode=Unused parameter value
  Upsample 1 : dspsigops/Upsample  N=2  phase=0  RateOptions=Allow multirate processing  ic=0  mode=Unused parameter value
  Upsample 2 : dspsigops/Upsample  N=2  phase=0  RateOptions=Allow multirate processing  ic=0  mode=Unused parameter value
  Out1 : Outport
  wires:
  Upsample/1 -> Delay/1
  Delay5/1 -> Sum6/2
  Add2/1 -> E7/1(In1), E6/1(In1), E5/1(In1), E4/1(In1), E3/1(In1), E2/1(In1), E1/1(In1), E0/1(In1)
  Upsample6/1 -> Sum6/1
  Delay4/1 -> Sum5/2
  Delay3/1 -> Sum4/2
  E5/1(Out1) -> Upsample2/1
  Sum6/1 -> Delay6/1
  Sum7/1 -> Delay1/1
  E7/1(Out1) -> Upsample/1
  Upsample1/1 -> Sum7/1
  Upsample2/1 -> Sum1/1
  Input/1 -> E1(Z)/1(Input1), E0(Z)/1(Input)
  E0(Z)/1(Out1) -> Upsample 1/1
  Upsample 2/1 -> Delay11/1
  Delay6/1 -> Sum8/2
  E0/1(Out1) -> Upsample7/1
  Delay/1 -> Sum7/2
  E1/1(Out1) -> Upsample6/1
  Delay1/1 -> Sum1/2
  Sum5/1 -> Delay5/1
  Sum4/1 -> Delay4/1
  Upsample5/1 -> Sum5/1
  Upsample 1/1 -> Add2/1
  Sum8/1 -> Out1/1
  Upsample4/1 -> Sum4/1
  Delay11/1 -> Add2/2
  Sum1/1 -> Delay2/1
  Sum2/1 -> Delay3/1
  E6/1(Out1) -> Upsample1/1
  E3/1(Out1) -> Upsample4/1
  Delay2/1 -> Sum2/2
  Upsample7/1 -> Sum8/1
  E1(Z)/1(Output) -> Upsample 2/1
  Upsample3/1 -> Sum2/1
  E2/1(Out1) -> Upsample5/1
  E4/1(Out1) -> Upsample3/1

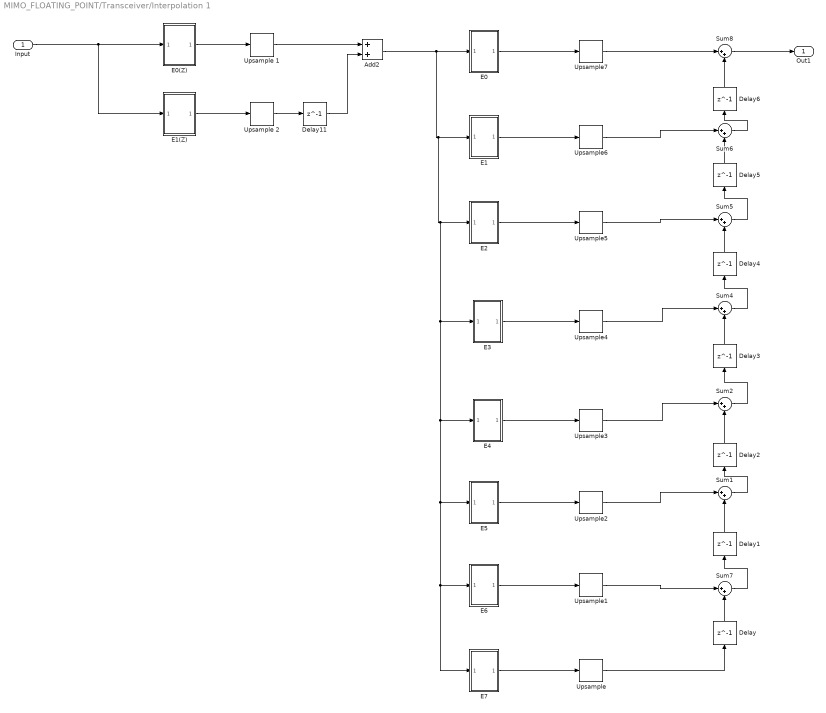
== system MIMO_FLOATING_POINT/Transceiver/Interpolation 1 ==
  Input : Inport
  Add2 : Sum
  Delay{,1..6,11} (8 alike) : Delay  DelayLength=1
  E0 : Subsystem
  E0(Z) : Subsystem
  E1 : Subsystem
  E1(Z) : Subsystem
  E2 : Subsystem
  E3 : Subsystem
  E4 : Subsystem
  E5 : Subsystem
  E6 : Subsystem
  E7 : Subsystem
  Sum{1..2,4..8} (7 alike) : Sum  Inputs=|++
  Upsample{,1..7} (8 alike) : dspsigops/Upsample  N=8  phase=0  RateOptions=Allow multirate processing  ic=0  mode=Unused parameter value
  Upsample 1 : dspsigops/Upsample  N=2  phase=0  RateOptions=Allow multirate processing  ic=0  mode=Unused parameter value
  Upsample 2 : dspsigops/Upsample  N=2  phase=0  RateOptions=Allow multirate processing  ic=0  mode=Unused parameter value
  Out1 : Outport
  wires:
  Upsample/1 -> Delay/1
  Delay5/1 -> Sum6/2
  Add2/1 -> E7/1(In1), E6/1(In1), E5/1(In1), E4/1(In1), E3/1(In1), E2/1(In1), E1/1(In1), E0/1(In1)
  Upsample6/1 -> Sum6/1
  Delay4/1 -> Sum5/2
  Delay3/1 -> Sum4/2
  E5/1(Out1) -> Upsample2/1
  Sum6/1 -> Delay6/1
  Sum7/1 -> Delay1/1
  E7/1(Out1) -> Upsample/1
  Upsample1/1 -> Sum7/1
  Upsample2/1 -> Sum1/1
  Input/1 -> E1(Z)/1(Input1), E0(Z)/1(Input)
  E0(Z)/1(Out1) -> Upsample 1/1
  Upsample 2/1 -> Delay11/1
  Delay6/1 -> Sum8/2
  E0/1(Out1) -> Upsample7/1
  Delay/1 -> Sum7/2
  E1/1(Out1) -> Upsample6/1
  Delay1/1 -> Sum1/2
  Sum5/1 -> Delay5/1
  Sum4/1 -> Delay4/1
  Upsample5/1 -> Sum5/1
  Upsample 1/1 -> Add2/1
  Sum8/1 -> Out1/1
  Upsample4/1 -> Sum4/1
  Delay11/1 -> Add2/2
  Sum1/1 -> Delay2/1
  Sum2/1 -> Delay3/1
  E6/1(Out1) -> Upsample1/1
  E3/1(Out1) -> Upsample4/1
  Delay2/1 -> Sum2/2
  Upsample7/1 -> Sum8/1
  E1(Z)/1(Output) -> Upsample 2/1
  Upsample3/1 -> Sum2/1
  E2/1(Out1) -> Upsample5/1
  E4/1(Out1) -> Upsample3/1

== system MIMO_FLOATING_POINT/Transceiver/Subsystem ==
  In1 : Inport
  Delay{,1,4..9} (8 alike) : Delay  DelayLength=1
  Delay2 : Delay  DelayLength=5
  Delay3 : Delay  DelayLength=3
  Gain : Gain
  Gain1 : Gain
  Gain2 : Gain
  Quantizer : Quantizer  QuantizationInterval=1
  Quantizer1 : Quantizer  QuantizationInterval=1
  Quantizer2 : Quantizer  QuantizationInterval=1
  Subtract : Sum  Inputs=+-
  Subtract1 : Sum  Inputs=+-
  Subtract2 : Sum  Inputs=+-
  Sum{,1..2,4,6} (5 alike) : Sum  Inputs=|++
  Sum3 : Sum  Inputs=|+-
  Sum5 : Sum  Inputs=|+-
  Out1 : Outport
  wires:
  Delay/1 -> Sum1/1, Gain/1
  Quantizer/1 -> Subtract/2, Delay2/1
  Sum/1 -> Subtract/1, Quantizer/1
  Sum2/1 -> Subtract2/1, Quantizer2/1
  Delay4/1 -> Gain2/1
  Delay8/1 -> Sum5/2
  Sum4/1 -> Sum5/1, Delay8/1
  Subtract/1 -> Delay/1
  Delay5/1 -> Delay6/1, Sum3/1
  Quantizer1/1 -> Subtract1/2, Delay3/1
  Delay1/1 -> Sum2/1, Gain1/1
  Gain2/1 -> Sum2/2
  Sum1/1 -> Subtract1/1, Quantizer1/1
  Subtract1/1 -> Delay1/1
  Gain1/1 -> Sum1/2
  Sum3/1 -> Delay7/1
  Gain/1 -> Sum/2
  Delay3/1 -> Sum4/1
  Delay7/1 -> Sum4/2
  Subtract2/1 -> Delay4/1
  Quantizer2/1 -> Subtract2/2, Delay5/1
  Delay6/1 -> Sum3/2
  Sum5/1 -> Delay9/1
  Delay2/1 -> Sum6/1
  Delay9/1 -> Sum6/2
  In1/1 -> Sum/1
  Sum6/1 -> Out1/1

== system MIMO_FLOATING_POINT/Transceiver/Subsystem1 ==
  In1 : Inport
  Delay{,1,4..9} (8 alike) : Delay  DelayLength=1
  Delay2 : Delay  DelayLength=5
  Delay3 : Delay  DelayLength=3
  Gain : Gain
  Gain1 : Gain
  Gain2 : Gain
  Quantizer : Quantizer  QuantizationInterval=1
  Quantizer1 : Quantizer  QuantizationInterval=1
  Quantizer2 : Quantizer  QuantizationInterval=1
  Subtract : Sum  Inputs=+-
  Subtract1 : Sum  Inputs=+-
  Subtract2 : Sum  Inputs=+-
  Sum{,1..2,4,6} (5 alike) : Sum  Inputs=|++
  Sum3 : Sum  Inputs=|+-
  Sum5 : Sum  Inputs=|+-
  Out1 : Outport
  wires:
  Delay/1 -> Sum1/1, Gain/1
  Quantizer/1 -> Subtract/2, Delay2/1
  Sum/1 -> Subtract/1, Quantizer/1
  Sum2/1 -> Subtract2/1, Quantizer2/1
  Delay4/1 -> Gain2/1
  Delay8/1 -> Sum5/2
  Sum4/1 -> Sum5/1, Delay8/1
  Subtract/1 -> Delay/1
  Delay5/1 -> Delay6/1, Sum3/1
  Quantizer1/1 -> Subtract1/2, Delay3/1
  Delay1/1 -> Sum2/1, Gain1/1
  Gain2/1 -> Sum2/2
  Sum1/1 -> Subtract1/1, Quantizer1/1
  Subtract1/1 -> Delay1/1
  Gain1/1 -> Sum1/2
  Sum3/1 -> Delay7/1
  Gain/1 -> Sum/2
  Delay3/1 -> Sum4/1
  Delay7/1 -> Sum4/2
  Subtract2/1 -> Delay4/1
  Quantizer2/1 -> Subtract2/2, Delay5/1
  Delay6/1 -> Sum3/2
  Sum5/1 -> Delay9/1
  Delay2/1 -> Sum6/1
  Delay9/1 -> Sum6/2
  In1/1 -> Sum/1
  Sum6/1 -> Out1/1

== system MIMO_FLOATING_POINT/Transceiver5/ADC 1 ==
  In1 : Inport
  SigmaDelta ADC : Subsystem
  Switch : Switch  Criteria=u2 > Threshold  SaturateOnIntegerOverflow=off  InputSameDT=off
  Zero : Constant  Value=0
  bits 1&0 : Outport
  wires:
  SigmaDelta ADC/1(Out) -> Switch/1, Switch/2
  Zero/1 -> Switch/3
  In1/1 -> SigmaDelta ADC/1(In)
  Switch/1 -> bits 1&0/1

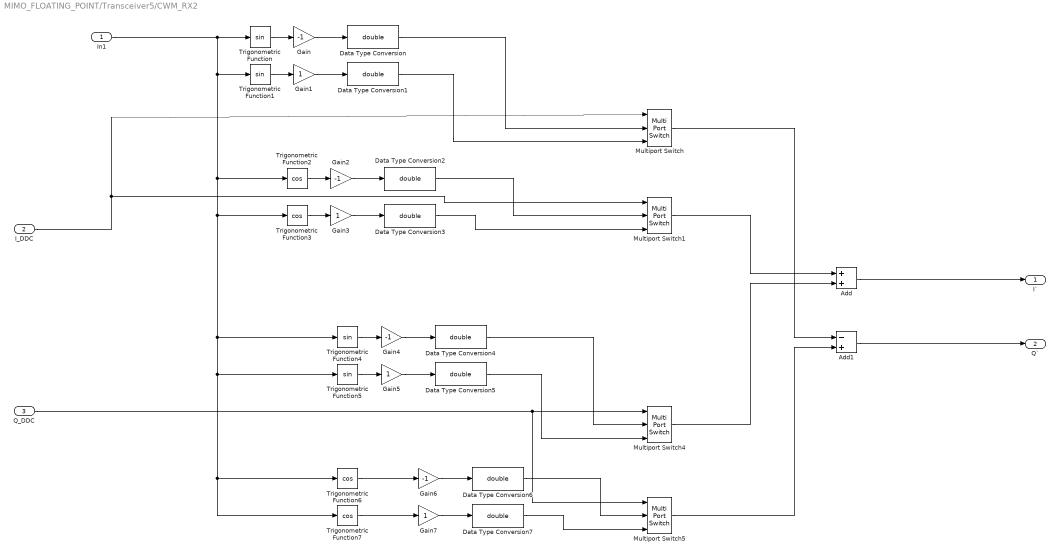
== system MIMO_FLOATING_POINT/Transceiver5/CWM_RX2 ==
  In1 : Inport
  I_DDC : Inport  Port=2
  Q_DDC : Inport  Port=3
  Add : Sum
  Add1 : Sum  Inputs=-+
  Data Type Conversion{,1..7} (8 alike) : DataTypeConversion  OutMin=-1  OutMax=1  OutDataTypeStr=double  RndMeth=Nearest
  Gain{,2,4,6} (4 alike) : Gain  Gain=-1
  Gain{1,3,5,7} (4 alike) : Gain
  Multiport Switch{,1,4..5} (4 alike) : MultiPortSwitch  DataPortOrder=Zero-based contiguous  Inputs=2  zeroidx=on  RndMeth=Nearest  SaturateOnIntegerOverflow=off  InputSameDT=off
  Trigonometric Function{,1,4..5} (4 alike) : Trigonometry
  Trigonometric Function{2..3,6..7} (4 alike) : Trigonometry  Operator=cos
  I` : Outport
  Q` : Outport  Port=2
  wires:
  Multiport Switch/1 -> Add1/1
  Add/1 -> I`/1
  I_DDC/1 -> Multiport Switch1/1, Multiport Switch/1
  Gain2/1 -> Data Type Conversion2/1
  Trigonometric Function5/1 -> Gain5/1
  Data Type Conversion2/1 -> Multiport Switch1/2
  Data Type Conversion1/1 -> Multiport Switch/3
  Gain5/1 -> Data Type Conversion5/1
  Gain4/1 -> Data Type Conversion4/1
  Trigonometric Function1/1 -> Gain1/1
  Data Type Conversion6/1 -> Multiport Switch5/2
  Gain1/1 -> Data Type Conversion1/1
  Gain3/1 -> Data Type Conversion3/1
  Trigonometric Function3/1 -> Gain3/1
  Add1/1 -> Q`/1
  Gain/1 -> Data Type Conversion/1
  Trigonometric Function2/1 -> Gain2/1
  In1/1 -> Trigonometric Function3/1, Trigonometric Function4/1, Trigonometric Function5/1, Trigonometric Function6/1, Trigonometric Function7/1, Trigonometric Function2/1, Trigonometric Function1/1, Trigonometric Function/1
  Q_DDC/1 -> Multiport Switch5/1, Multiport Switch4/1
  Data Type Conversion7/1 -> Multiport Switch5/3
  Data Type Conversion4/1 -> Multiport Switch4/2
  Trigonometric Function6/1 -> Gain6/1
  Gain7/1 -> Data Type Conversion7/1
  Trigonometric Function4/1 -> Gain4/1
  Trigonometric Function/1 -> Gain/1
  Multiport Switch1/1 -> Add/1
  Multiport Switch4/1 -> Add/2
  Trigonometric Function7/1 -> Gain7/1
  Multiport Switch5/1 -> Add1/2
  Data Type Conversion5/1 -> Multiport Switch4/3
  Gain6/1 -> Data Type Conversion6/1
  Data Type Conversion/1 -> Multiport Switch/2
  Data Type Conversion3/1 -> Multiport Switch1/3

== system MIMO_FLOATING_POINT/Transceiver5/CWM_TX_Chain_1 ==
  PHI : Inport
  Processor_I : Inport  Port=2
  Processor_Q : Inport  Port=3
  Add : Sum  OutDataTypeStr=double  RndMeth=Round  SaturateOnIntegerOverflow=on
  Add1 : Sum  OutDataTypeStr=double
  Data Type Conversion{1..4} (4 alike) : DataTypeConversion  Commented=through  OutMin=-1  OutMax=1  OutDataTypeStr=fixdt(1,8,6)  RndMeth=Nearest
  Gain1 : Gain  Gain=-1
  Gain2 : Gain
  Gain3 : Gain
  Gain4 : Gain
  Hamming : Gain  OutDataTypeStr=double
  Hamming1 : Gain  OutDataTypeStr=double
  Product{,1..3} (4 alike) : Product
  Trigonometric Function1 : Trigonometry
  Trigonometric Function2 : Trigonometry  Operator=cos
  Trigonometric Function3 : Trigonometry  Operator=cos
  Trigonometric Function4 : Trigonometry
  I_1 : Outport
  Q_1 : Outport  Port=2
  wires:
  Trigonometric Function2/1 -> Gain2/1
  Gain2/1 -> Data Type Conversion2/1
  Processor_Q/1 -> Product1/2, Product3/2
  Processor_I/1 -> Product2/1, Product/1
  Gain1/1 -> Data Type Conversion1/1
  Product/1 -> Add/1
  Trigonometric Function1/1 -> Gain1/1
  PHI/1 -> Trigonometric Function2/1, Trigonometric Function1/1, Trigonometric Function4/1, Trigonometric Function3/1
  Data Type Conversion1/1 -> Product1/1
  Gain3/1 -> Data Type Conversion3/1
  Product2/1 -> Add1/1
  Data Type Conversion2/1 -> Product/2
  Data Type Conversion4/1 -> Product2/2
  Data Type Conversion3/1 -> Product3/1
  Product3/1 -> Add1/2
  Trigonometric Function3/1 -> Gain3/1
  Product1/1 -> Add/2
  Gain4/1 -> Data Type Conversion4/1
  Trigonometric Function4/1 -> Gain4/1
  Add/1 -> Hamming/1
  Add1/1 -> Hamming1/1
  Hamming/1 -> I_1/1
  Hamming1/1 -> Q_1/1

== system MIMO_FLOATING_POINT/Transceiver5/DDC2 ==
  ODD_I : Inport
  EVEN_Q : Inport  Port=2
  Local_Oscilator1 : DiscretePulseGenerator  PhaseDelay=1  SampleTime=0.02
  Logical Operator : Logic  Operator=NXOR  AllPortsSameDT=off  OutDataTypeStr=boolean
  Logical Operator1 : Logic  Operator=NXOR  AllPortsSameDT=off  OutDataTypeStr=boolean
  NOT : Logic  Operator=NOT  IconShape=distinctive  AllPortsSameDT=off  OutDataTypeStr=boolean
  Scope1 : Scope  NumInputPorts=3
  Scope2 : Scope  NumInputPorts=3
  I_DDC : Outport
  Q_DDC : Outport  Port=2
  wires:
  Logical Operator/1 -> Scope2/3, I_DDC/1
  EVEN_Q/1 -> Scope1/1, Logical Operator1/2
  ODD_I/1 -> Scope2/1, Logical Operator/1
  Logical Operator1/1 -> Scope1/3, Q_DDC/1
  Local_Oscilator1/1 -> NOT/1
  NOT/1 -> Scope1/2, Logical Operator1/1, Scope2/2, Logical Operator/2

== system MIMO_FLOATING_POINT/Transceiver5/DUC2 ==
  I_1 : Inport
  Q_1 : Inport  Port=2
  -cos : Sin  SineType=Sample based  Frequency=2*pi*100  Phase=pi/2  Samples=4  SampleTime=0.01  Offset=3
  -sin1 : Sin  SineType=Sample based  Frequency=(2*pi*100)/4  Samples=4  SampleTime=.01  Offset=2
  Add : Sum
  Constant : Constant  Value=0
  Constant1 : Constant  Value=0
  Gain : Gain  Gain=-1
  Gain1 : Gain  Gain=-1
  Multiport Switch : MultiPortSwitch  DataPortOrder=Specify indices  DataPortIndices={1,0,-1}  RndMeth=Nearest  SaturateOnIntegerOverflow=off  InputSameDT=off
  Multiport Switch1 : MultiPortSwitch  DataPortOrder=Specify indices  DataPortIndices={1,0,-1}  RndMeth=Nearest  SaturateOnIntegerOverflow=off  InputSameDT=off
  Scope : Scope  NumInputPorts=3
  Scope1 : Scope  NumInputPorts=3
  Scope2 : Scope  NumInputPorts=3
  Out2 : Outport
  wires:
  Constant/1 -> Multiport Switch1/3
  Q_1/1 -> Gain1/1, Multiport Switch/2, Scope/1
  I_1/1 -> Gain/1, Scope2/1, Multiport Switch1/2
  Gain1/1 -> Multiport Switch/4
  -sin1/1 -> Scope/2, Multiport Switch/1
  -cos/1 -> Scope2/2, Multiport Switch1/1
  Multiport Switch/1 -> Scope/3, Scope1/2, Add/2
  Add/1 -> Scope1/3, Out2/1
  Multiport Switch1/1 -> Add/1, Scope1/1, Scope2/3
  Constant1/1 -> Multiport Switch/3
  Gain/1 -> Multiport Switch1/4

== system MIMO_FLOATING_POINT/Transceiver5/Inter_Lever2 ==
  bits 1&0 : Inport
  Delay1 : Delay  DelayLength=1  InitialCondition=0
  Delay2 : Delay  DelayLength=1  InitialCondition=0
  Downsample : DownSample  RateOptions=Allow multirate processing
  Downsample1 : DownSample  RateOptions=Allow multirate processing
  Scope1 : Scope  NumInputPorts=3
  ODD_I : Outport
  EVEN_Q : Outport  Port=2
  wires:
  Delay1/1 -> Downsample1/1
  Downsample/1 -> Delay2/1
  Downsample1/1 -> Scope1/3, EVEN_Q/1
  bits 1&0/1 -> Scope1/1, Delay1/1, Downsample/1
  Delay2/1 -> Scope1/2, ODD_I/1

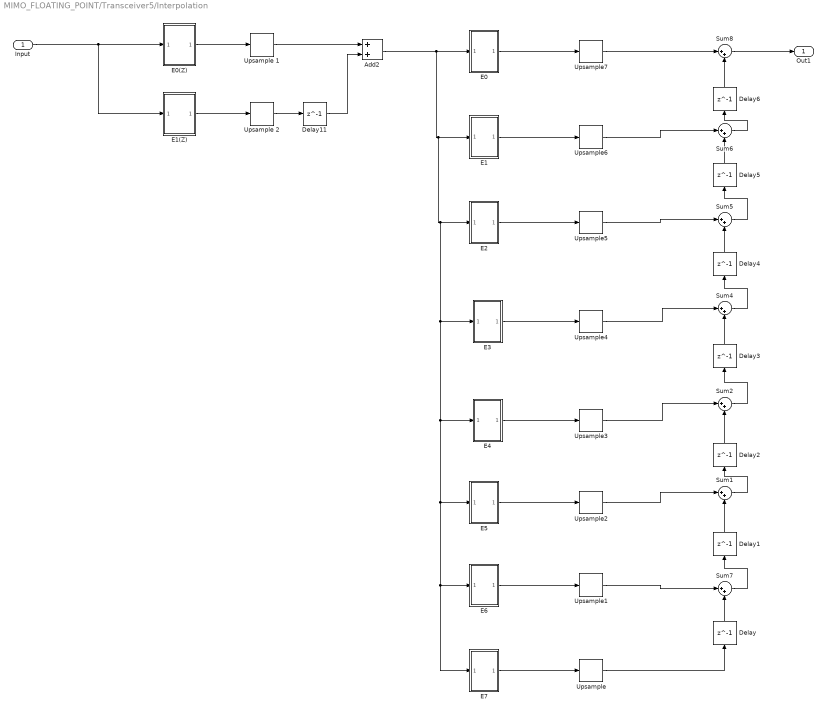
== system MIMO_FLOATING_POINT/Transceiver5/Interpolation  ==
  Input : Inport
  Add2 : Sum
  Delay{,1..6,11} (8 alike) : Delay  DelayLength=1
  E0 : Subsystem
  E0(Z) : Subsystem
  E1 : Subsystem
  E1(Z) : Subsystem
  E2 : Subsystem
  E3 : Subsystem
  E4 : Subsystem
  E5 : Subsystem
  E6 : Subsystem
  E7 : Subsystem
  Sum{1..2,4..8} (7 alike) : Sum  Inputs=|++
  Upsample{,1..7} (8 alike) : dspsigops/Upsample  N=8  phase=0  RateOptions=Allow multirate processing  ic=0  mode=Unused parameter value
  Upsample 1 : dspsigops/Upsample  N=2  phase=0  RateOptions=Allow multirate processing  ic=0  mode=Unused parameter value
  Upsample 2 : dspsigops/Upsample  N=2  phase=0  RateOptions=Allow multirate processing  ic=0  mode=Unused parameter value
  Out1 : Outport
  wires:
  Upsample/1 -> Delay/1
  Delay5/1 -> Sum6/2
  Add2/1 -> E7/1(In1), E6/1(In1), E5/1(In1), E4/1(In1), E3/1(In1), E2/1(In1), E1/1(In1), E0/1(In1)
  Upsample6/1 -> Sum6/1
  Delay4/1 -> Sum5/2
  Delay3/1 -> Sum4/2
  E5/1(Out1) -> Upsample2/1
  Sum6/1 -> Delay6/1
  Sum7/1 -> Delay1/1
  E7/1(Out1) -> Upsample/1
  Upsample1/1 -> Sum7/1
  Upsample2/1 -> Sum1/1
  Input/1 -> E1(Z)/1(Input1), E0(Z)/1(Input)
  E0(Z)/1(Out1) -> Upsample 1/1
  Upsample 2/1 -> Delay11/1
  Delay6/1 -> Sum8/2
  E0/1(Out1) -> Upsample7/1
  Delay/1 -> Sum7/2
  E1/1(Out1) -> Upsample6/1
  Delay1/1 -> Sum1/2
  Sum5/1 -> Delay5/1
  Sum4/1 -> Delay4/1
  Upsample5/1 -> Sum5/1
  Upsample 1/1 -> Add2/1
  Sum8/1 -> Out1/1
  Upsample4/1 -> Sum4/1
  Delay11/1 -> Add2/2
  Sum1/1 -> Delay2/1
  Sum2/1 -> Delay3/1
  E6/1(Out1) -> Upsample1/1
  E3/1(Out1) -> Upsample4/1
  Delay2/1 -> Sum2/2
  Upsample7/1 -> Sum8/1
  E1(Z)/1(Output) -> Upsample 2/1
  Upsample3/1 -> Sum2/1
  E2/1(Out1) -> Upsample5/1
  E4/1(Out1) -> Upsample3/1
